simulink model "dynamiczny_model_dyskretny"  (R2021a)
settings: Solver=VariableStepAuto  StartTime=0.0  StopTime=10.0  RelTol=1e-3
values from neighbouring files (symbols this model uses):
  T = 0.5    [z3_czas_probkowania_T.m]    (also in z9_czas_probkowania_T_wartosc_ud.m = 1)
settings Model: Creator=48604  LastModifiedBy=48604

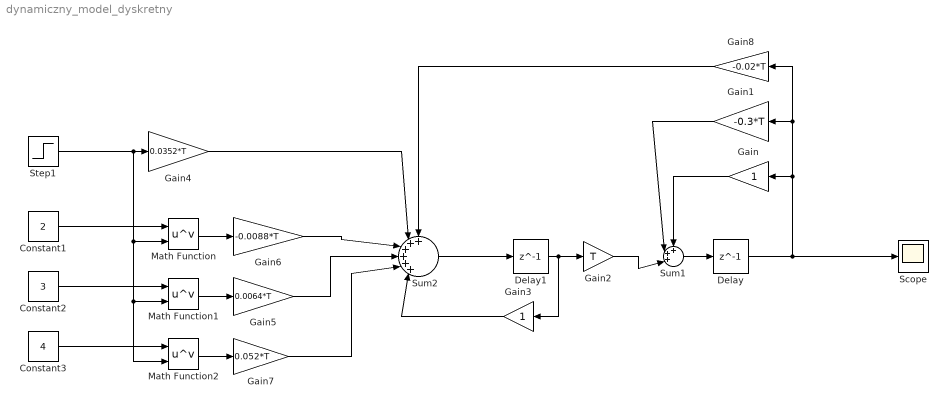
== system dynamiczny_model_dyskretny ==
  Constant1 : Constant  Value=2
  Constant2 : Constant  Value=3
  Constant3 : Constant  Value=4
  Delay : Delay  DelayLength=1  InitialCondition=0
  Delay1 : Delay  DelayLength=1  InitialCondition=0
  Gain : Gain
  Gain1 : Gain  Gain=-0.3*T
  Gain2 : Gain  Gain=T
  Gain3 : Gain
  Gain4 : Gain  Gain=0.0352*T
  Gain5 : Gain  Gain=0.0064*T
  Gain6 : Gain  Gain=-0.0088*T
  Gain7 : Gain  Gain=0.052*T
  Gain8 : Gain  Gain=-0.02*T
  Math Function : Math  Operator=pow  SaturateOnIntegerOverflow=on
  Math Function1 : Math  Operator=pow  SaturateOnIntegerOverflow=on
  Math Function2 : Math  Operator=pow  SaturateOnIntegerOverflow=on
  Scope : Scope
  Step1 : Step  SampleTime=0.5
  Sum1 : Sum  Inputs=+++|
  Sum2 : Sum  Inputs=++++++|
  wires:
  Sum1/1 -> Delay/1
  Delay/1 -> Gain1/1, Gain8/1, Gain/1, Scope/1
  Gain/1 -> Sum1/1
  Gain1/1 -> Sum1/2
  Gain2/1 -> Sum1/3
  Delay1/1 -> Gain3/1, Gain2/1
  Step1/1 -> Math Function2/2, Math Function1/2, Math Function/2, Gain4/1
  Gain4/1 -> Sum2/2
  Math Function/1 -> Gain6/1
  Math Function1/1 -> Gain5/1
  Constant2/1 -> Math Function1/1
  Gain6/1 -> Sum2/3
  Gain5/1 -> Sum2/4
  Gain7/1 -> Sum2/5
  Constant1/1 -> Math Function/1
  Constant3/1 -> Math Function2/1
  Math Function2/1 -> Gain7/1
  Sum2/1 -> Delay1/1
  Gain3/1 -> Sum2/6
  Gain8/1 -> Sum2/1
